simulink model "simpleModel"  (R2023a)
settings: Solver=VariableStepAuto  StartTime=0.0  StopTime=10.0  RelTol=1e-3
settings Model: Creator=neham  LastModifiedBy=neham

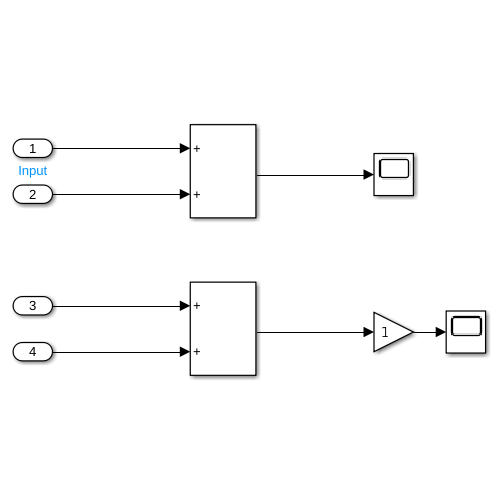
[thumbnail: Simulink's stored preview of the top-level diagram]
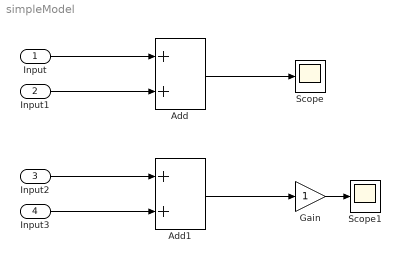
== system simpleModel ==
  Input : Inport
  Input1 : Inport  Port=2
  Input2 : Inport  Port=3
  Input3 : Inport  Port=4
  Add : Sum
  Add1 : Sum
  Gain : Gain
  Scope : Scope
  Scope1 : Scope
  wires:
  Input/1 -> Add/1
  Input1/1 -> Add/2
  Add/1 -> Scope/1
  Input2/1 -> Add1/1
  Input3/1 -> Add1/2
  Add1/1 -> Gain/1
  Gain/1 -> Scope1/1
